simulink model "TrimPlane"  (R2021a)
settings: Solver=ode23t  StartTime=0.0  StopTime=5000  RelTol=1e-3
undefined symbols (not defined in the file or in its folder): F, MIL, Moderate, plane
libraries: aerolibasang x2, shared6dof x1, sharedtransform x1, aerolibadyn x1, aerolibwind2 x1, aerolibatmos2 x1
settings Model: Creator=janbe  LastModifiedBy=janbe

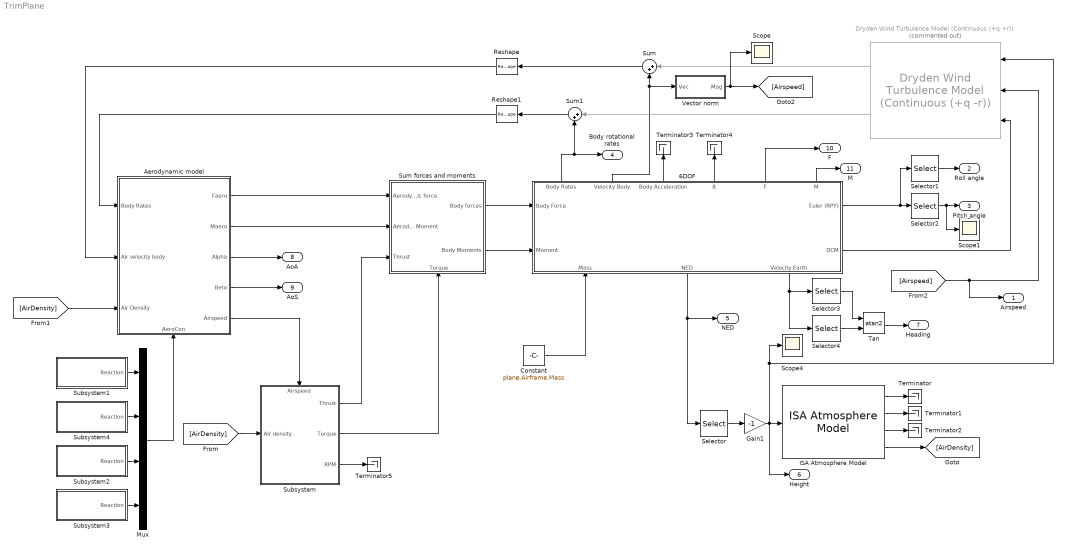
== system TrimPlane ==
  6DOF : Subsystem
      settings: PortSchema="{\"entries\":[{\"content\":{\"sides\":[{\"content\":{\"connectorIds\":[\"In1\",\"In2\"]},\"type\":\"ConnectorPlacement.EquallySpacedRectSide\",\"uuid\":\"48c1bbec-9b7a-4998-8085-77477050d4c3\"},{\"content\":{\"connectorIds\":[\"Out1\",\"Out2\"],\"side\":\"RIGHT\"},\"type\":\"ConnectorPlacement.EquallySpacedRectSide\",\"uuid\":\"5fc5dd37-324a-470e-bd5f-bf29eb3f91cd\"},{\"content\":{\"connectorIds\":[\"Out5\",\"Out6\",\"Out7\",\"Out8\",\"Out9\",\"Out10\"],\"side\":\"TOP\"},\"type\":\"ConnectorPlacement.EquallySpacedRectSide\",\"uuid\":\"ad20a820-91fa-4a98-9c09-942563c80c3d\"},{\"content\":{\"connectorIds\":[\"In3\",\"Out3\",\"Out4\"],\"side\":\"BOTTOM\"},\"type\":\"ConnectorPlacement.EquallySpacedRectSide\",\"uuid\":\"0b972b14-3415-44ab-ae5c-f6c492f3b9a5\"}]},\"type\":\"ConnectorPlacement.EquallySpacedConnector\",\"uuid\":\"3b00a1ae-2557-41be-80c2-23bcdc8281c3\"}],\"packageUris\":[\"http://schema.mathworks.com/mf0/Connector/R2020b\"],\"version\":\"1.0\"}"
  Aerodynamic model : Subsystem
      settings: PortSchema="{\"entries\":[{\"content\":{\"sides\":[{\"content\":{\"connectorIds\":[\"In1\",\"In2\",\"In3\"]},\"type\":\"ConnectorPlacement.EquallySpacedRectSide\",\"uuid\":\"123ed6f9-c03c-44a2-9337-b402a98582dd\"},{\"content\":{\"connectorIds\":[\"Out1\",\"Out2\",\"Out3\",\"Out4\",\"Out5\"],\"side\":\"RIGHT\"},\"type\":\"ConnectorPlacement.EquallySpacedRectSide\",\"uuid\":\"6aca0a3c-b214-45a7-a9f0-b8fb94350ea4\"},{\"content\":{\"connectorIds\":[],\"side\":\"TOP\"},\"type\":\"ConnectorPlacement.EquallySpacedRectSide\",\"uuid\":\"093f64cd-11d7-4128-9556-c22df5842c81\"},{\"content\":{\"connectorIds\":[\"In4\"],\"side\":\"BOTTOM\"},\"type\":\"ConnectorPlacement.EquallySpacedRectSide\",\"uuid\":\"6978f55d-1ae4-4dbf-af4a-386a3019c4ac\"}]},\"type\":\"ConnectorPlacement.EquallySpacedConnector\",\"uuid\":\"655dc0fe-ac89-4e4b-af89-368bfcff1c7c\"}],\"packageUris\":[\"http://schema.mathworks.com/mf0/Connector/R2020b\"],\"version\":\"1.0\"}"
  Constant : Constant  Value=plane.Airframe.Mass
  Dryden Wind Turbulence Model (Continuous (+q +r)) : aerolibwind2/Dryden Wind Turbulence Model  (Continuous (+q -r))  Commented=on  units=Metric (MKS)  spec=MIL-F-8785C  model=Continuous Von Karman (+q -r)  W20=15  Wdeg=0  TurbProb=10^-3 - Moderate  L_high=533.4  Wingspan=19.478  ts=0.1  Seed=[23341 23342 23343 23344]  T_on=off
  Gain1 : Gain  Gain=-1
  ISA Atmosphere Model : aerolibatmos2/ISA Atmosphere Model  custom=off  g=9.80665  gamma=1.4  R=287.0531  L=0.0065  h_trop=11000  h_strat=20000  rho0=1.225  P0=101325  T0=288.15  h0=0
  Mux : Mux
  Reshape : Reshape  OutputDimensionality=Column vector (2-D)
  Reshape1 : Reshape  OutputDimensionality=Column vector (2-D)
  Scope : Scope
  Scope1 : Scope
  Scope4 : Scope
  Selector : Selector  InputPortWidth=3  IndexOptions=Index vector (dialog)  Indices=3  OutputSizes=1
  Selector1 : Selector  InputPortWidth=3  IndexOptions=Index vector (dialog)  Indices=1  OutputSizes=1
  Selector2 : Selector  InputPortWidth=3  IndexOptions=Index vector (dialog)  Indices=2  OutputSizes=1
  Selector3 : Selector  InputPortWidth=3  IndexOptions=Index vector (dialog)  Indices=2  OutputSizes=1
  Selector4 : Selector  InputPortWidth=3  IndexOptions=Index vector (dialog)  Indices=1  OutputSizes=1
  Subsystem : Subsystem
      settings: PortSchema="{\"entries\":[{\"content\":{\"sides\":[{\"content\":{\"connectorIds\":[\"In1\"]},\"type\":\"ConnectorPlacement.EquallySpacedRectSide\",\"uuid\":\"8b318bb3-5013-4f5e-bd3e-2f5669bf6358\"},{\"content\":{\"connectorIds\":[\"Out1\",\"Out2\",\"Out3\"],\"side\":\"RIGHT\"},\"type\":\"ConnectorPlacement.EquallySpacedRectSide\",\"uuid\":\"500402ef-b296-45ac-a743-b1e2b9e33679\"},{\"content\":{\"connectorIds\":[\"In2\"],\"side\":\"TOP\"},\"type\":\"ConnectorPlacement.EquallySpacedRectSide\",\"uuid\":\"5cfe175c-55a3-4920-8fe6-6fd8cc9eed8d\"}]},\"type\":\"ConnectorPlacement.EquallySpacedConnector\",\"uuid\":\"49d65523-413b-4dcb-9879-1a0370ab7ce2\"}],\"packageUris\":[\"http://schema.mathworks.com/mf0/Connector/R2020b\"],\"version\":\"1.0\"}"
  Subsystem1 : Subsystem
  Subsystem2 : Subsystem
  Subsystem3 : Subsystem
  Subsystem4 : Subsystem
  Sum : Sum  Inputs=|++
  Sum forces and moments : Subsystem
      settings: PortSchema="{\"entries\":[{\"content\":{\"sides\":[{\"content\":{\"connectorIds\":[\"In1\",\"In2\",\"In3\"]},\"type\":\"ConnectorPlacement.EquallySpacedRectSide\",\"uuid\":\"38dc5884-e381-4ee1-b666-063f48dc30b0\"},{\"content\":{\"connectorIds\":[\"Out1\",\"Out2\"],\"side\":\"RIGHT\"},\"type\":\"ConnectorPlacement.EquallySpacedRectSide\",\"uuid\":\"f2accc80-19db-41a7-90ee-23d63e2eaee3\"},{\"content\":{\"connectorIds\":[],\"side\":\"TOP\"},\"type\":\"ConnectorPlacement.EquallySpacedRectSide\",\"uuid\":\"1b11c4b8-c720-481f-9c75-f8744fb4ebda\"},{\"content\":{\"connectorIds\":[\"In4\"],\"side\":\"BOTTOM\"},\"type\":\"ConnectorPlacement.EquallySpacedRectSide\",\"uuid\":\"feccc13e-1f0d-4c40-950e-b0861e641184\"}]},\"type\":\"ConnectorPlacement.EquallySpacedConnector\",\"uuid\":\"fb9299ee-4c49-45c5-85b3-a138e0bb7e95\"}],\"packageUris\":[\"http://schema.mathworks.com/mf0/Connector/R2020b\"],\"version\":\"1.0\"}"
  Sum1 : Sum  Inputs=|++
  Tan : Trigonometry  Operator=atan2
  Terminator{,1..5} (6 alike) : Terminator
  Vector norm : Subsystem  mask(Vector norm-2){}
      mask help: Compute the 2-norm (magnitude) of a vector, |v| = sqrt(v'v).
      mask Help:
      | The block compute the 2-norm (or magnitude) of a vector.
      | <P><B>Input:</B> nx1 vector;</P>
      | <P><B>Output:</B> scalar magnitude.</P>
  Airspeed : Outport  Unit=m/s
  Roll angle : Outport  Port=2  Unit=rad
  Pitch angle : Outport  Port=3  Unit=rad
  Body rotational rates : Outport  Port=4  Unit=rad/s
  NED : Outport  Port=5  Unit=m
  Height : Outport  Port=6  Unit=m
  Heading : Outport  Port=7  Unit=rad
  AoA : Outport  Port=8  Unit=rad
  AoS : Outport  Port=9  Unit=rad
  F : Outport  Port=10
  M : Outport  Port=11
  wires:
  Aerodynamic model/2(Maero) -> Sum forces and moments/2(Aerodynamic Moment)
  6DOF/3(NED) -> Selector/1, NED/1
  Subsystem1/1(Reaction) -> Mux/1
  [AirDensity] -> Aerodynamic model/3(Air Density)
  [AirDensity] -> Subsystem/1(Air density)
  Selector2/1 -> Scope1/1, Pitch angle/1
  ISA Atmosphere Model/1 -> Terminator/1
  6DOF/2(DCM) -> Dryden Wind Turbulence Model (Continuous (+q +r))/3
  Dryden Wind Turbulence Model (Continuous (+q +r))/1 -> Sum/1
  Selector4/1 -> Tan/2
  Selector1/1 -> Roll angle/1
  ISA Atmosphere Model/4 -> [AirDensity]
  Vector norm/1(Mag) -> Scope/1, [Airspeed]
  Subsystem/3(RPM) -> Terminator5/1
  Aerodynamic model/4(Beta) -> AoS/1
  Tan/1 -> Heading/1
  Sum1/1 -> Reshape1/1
  Reshape1/1 -> Aerodynamic model/1(Body Rates)
  Constant/1 -> 6DOF/3(Mass)
  Subsystem4/1(Reaction) -> Mux/2
  6DOF/5(Body Rates) -> Body rotational rates/1, Sum1/2
  Subsystem2/1(Reaction) -> Mux/3
  6DOF/1(Euler (RPY)) -> Selector2/1, Selector1/1
  Sum/1 -> Reshape/1
  ISA Atmosphere Model/2 -> Terminator1/1
  Selector3/1 -> Tan/1
  Reshape/1 -> Aerodynamic model/2(Air velocity body)
  6DOF/6(Velocity Body) -> Vector norm/1(Vec), Sum/2
  Selector/1 -> Gain1/1
  Aerodynamic model/1(Faero) -> Sum forces and moments/1(Aerodynamic force)
  Aerodynamic model/3(Alpha) -> AoA/1
  Sum forces and moments/1(Body forces) -> 6DOF/1(Body Force)
  6DOF/4(Velocity Earth) -> Selector4/1, Selector3/1
  Sum forces and moments/2(Body Moments) -> 6DOF/2(Moment)
  Subsystem3/1(Reaction) -> Mux/4
  Dryden Wind Turbulence Model (Continuous (+q +r))/2 -> Sum1/1
  Mux/1 -> Aerodynamic model/4(AeroCon)
  Gain1/1 -> Height/1, Scope4/1, Dryden Wind Turbulence Model (Continuous (+q +r))/1, ISA Atmosphere Model/1
  [Airspeed] -> Airspeed/1, Dryden Wind Turbulence Model (Continuous (+q +r))/2
  ISA Atmosphere Model/3 -> Terminator2/1
  6DOF/8(Inertial Acceleration) -> Terminator4/1
  6DOF/7(Body Acceleration) -> Terminator3/1
  Aerodynamic model/5(Airspeed) -> Subsystem/2(Airspeed)
  Subsystem/1(Thrust) -> Sum forces and moments/3(Thrust)
  Subsystem/2(Torque) -> Sum forces and moments/4(Torque)
  6DOF/10(M) -> M/1
  6DOF/9(F) -> F/1

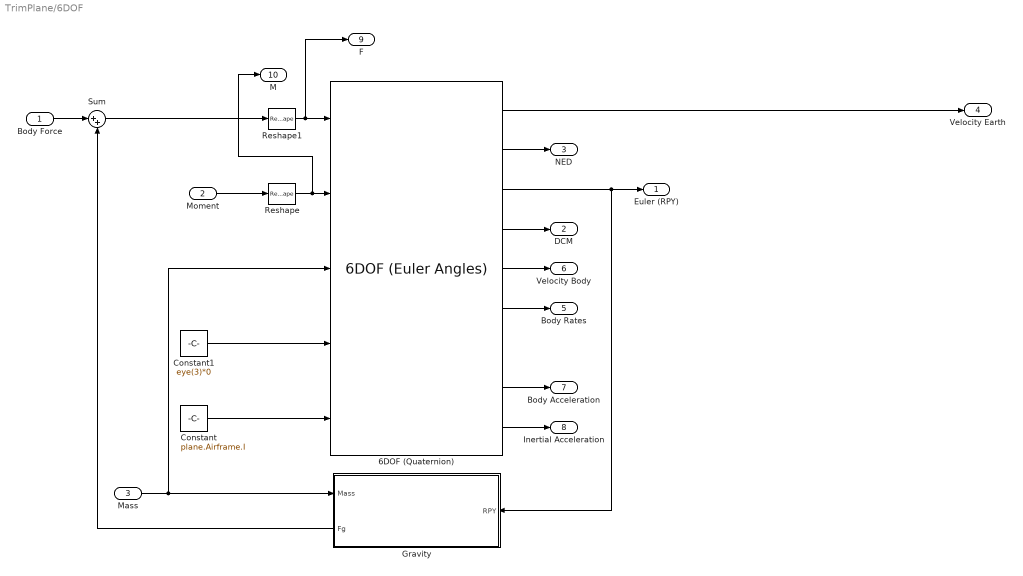
== system TrimPlane/6DOF ==
  Body Force : Inport  Unit=N  PortDimensions=[3 1]
  Moment : Inport  Port=2  Unit=N*m  PortDimensions=[3 1]
  Mass : Inport  Port=3  Unit=kg  PortDimensions=1
  6DOF (Quaternion) : shared6dof/6DOF (Euler Angles)  units=Metric (MKS)  mtype=Custom Variable  rep=Quaternion  xme_0=[0 0 -plane.trim.height]  Vm_0=plane.trim.BodyV  eul_0=[plane.trim.roll plane.trim.pitch 0]  pm_0=plane.trim.BodyRate  mass_0=1.0  mass_e=0.5  mass_f=2.0  inertia=eye(3)  inertia_e=eye(3)  inertia_f=2*eye(3)  k_quat=1.0  vre_flag=off  abi_flag=on  aMode=0  xme_statename=['North','East','Down']  Vm_statename=['Vx','Vy','Vz']  eul_statename=''  quat_statename=''  pm_statename=['Roll_rate_p','Pitch_rate_q','Yaw_rate_r']  mass_statename=''
      settings: SourceProductBaseCode=AE,PW,DR,MT,UV,VE
  Constant : Constant  Value=plane.Airframe.I
  Constant1 : Constant  Value=eye(3)*0
  Gravity : Subsystem
      settings: PortSchema="{\"entries\":[{\"content\":{\"sides\":[{\"content\":{\"connectorIds\":[\"In1\"]},\"type\":\"ConnectorPlacement.EquallySpacedRectSide\",\"uuid\":\"6f94d740-82bf-458e-8aa5-36b62f7e3ce2\"},{\"content\":{\"connectorIds\":[\"In2\",\"Out1\"],\"side\":\"RIGHT\"},\"type\":\"ConnectorPlacement.EquallySpacedRectSide\",\"uuid\":\"bdd5df12-d14f-445f-9bdc-a906ddbef1d8\"},{\"content\":{\"connectorIds\":[],\"side\":\"TOP\"},\"type\":\"ConnectorPlacement.EquallySpacedRectSide\",\"uuid\":\"cebee685-71c6-4366-9c39-37a9487371f5\"},{\"content\":{\"connectorIds\":[],\"side\":\"BOTTOM\"},\"type\":\"ConnectorPlacement.EquallySpacedRectSide\",\"uuid\":\"d1e10f76-8344-46b9-aae8-e8382cc28aaf\"}]},\"type\":\"ConnectorPlacement.EquallySpacedConnector\",\"uuid\":\"3d57e629-d59a-436c-b4c0-fcf54e0e0441\"}],\"packageUris\":[\"http://schema.mathworks.com/mf0/Connector/R2020b\"],\"version\":\"1.0\"}"
  Reshape : Reshape
  Reshape1 : Reshape
  Sum : Sum  Inputs=|++
  Euler (RPY) : Outport  Unit=rad
  DCM : Outport  Port=2
  NED : Outport  Port=3  Unit=m
  Velocity Earth : Outport  Port=4  Unit=m/s
  Body Rates : Outport  Port=5  Unit=rad/s
  Velocity Body : Outport  Port=6  Unit=m/s
  Body Acceleration : Outport  Port=7  Unit=m/s^2
  Inertial Acceleration : Outport  Port=8  Unit=m/s^2
  F : Outport  Port=9
  M : Outport  Port=10
  wires:
  6DOF (Quaternion)/5 -> Velocity Body/1
  6DOF (Quaternion)/3 -> Gravity/1(RPY), Euler (RPY)/1
  6DOF (Quaternion)/6 -> Body Rates/1
  6DOF (Quaternion)/8 -> Body Acceleration/1
  6DOF (Quaternion)/9 -> Inertial Acceleration/1
  6DOF (Quaternion)/1 -> Velocity Earth/1
  Mass/1 -> Gravity/2(Mass), 6DOF (Quaternion)/3
  Constant1/1 -> 6DOF (Quaternion)/4
  Reshape/1 -> M/1, 6DOF (Quaternion)/2
  Reshape1/1 -> F/1, 6DOF (Quaternion)/1
  6DOF (Quaternion)/2 -> NED/1
  Body Force/1 -> Sum/1
  Gravity/1(Fg) -> Sum/2
  Moment/1 -> Reshape/1
  Constant/1 -> 6DOF (Quaternion)/5
  Sum/1 -> Reshape1/1
  6DOF (Quaternion)/4 -> DCM/1

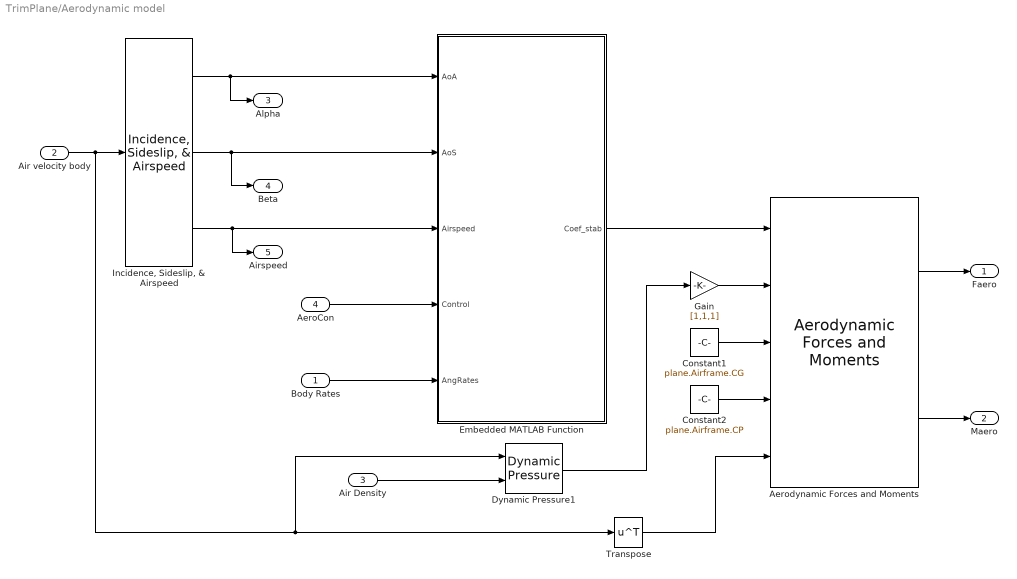
== system TrimPlane/Aerodynamic model ==
  Body Rates : Inport  Unit=rad/s  PortDimensions=[3 1]
  Air velocity body : Inport  Port=2  Unit=m/s  PortDimensions=[3 1]
  Air Density : Inport  Port=3  Unit=kg/m^3  PortDimensions=1
  AeroCon : Inport  Port=4  Unit=rad
  "Aerodynamic Forces and Moments " : aerolibadyn/Aerodynamic Forces and Moments   inputAxes=Stability  outputForceAxes=Body  outputMomentAxes=Body  S=plane.Airframe.A  b=plane.Airframe.S  cbar=plane.Airframe.MAC
  Constant1 : Constant  Value=plane.Airframe.CG
  Constant2 : Constant  Value=plane.Airframe.CP
  Dynamic Pressure1 : aerolibasang/Dynamic Pressure
  Embedded MATLAB Function : MATLAB Function  TreatAsAtomicUnit=on  mask{CL0=plane.Aerodynamic.CL0, dCLdAoA=plane.Aerodynamic.dCLdAoA, CD0=plane.Aerodynamic.CD0, CDmin=plane.Aerodynamic.CDmin, dCDdCL=plane.Aerodynamic.dCDdCL, dClAoS=plane.Aerodynamic.dClAoS, dClY=plane.Aerodynamic.dClY, dClP=plane.Aerodynamic.dClP, Cm0=plane.Aerodynamic.Cm0, dCmCL=plane.Aerodynamic.dCmCL, dCmQ=plane.Aerodynamic.dCmQ, dCnAoS=plane.Aerodynamic.CnAoS, dCnY=plane.Aerodynamic.dCnY, dCnP=plane.Aerodynamic.dCnP, C2M=plane.Aerodynamic.C2M, C2CL=plane.Aerodynamic.C2CL, C2CD=plane.Aerodynamic.C2CD}
  Gain : Gain  Gain=[1,1,1]
  "Incidence, Sideslip, & Airspeed" : aerolibasang/Incidence, Sideslip, & Airspeed
  Transpose : Math  Operator=transpose  SaturateOnIntegerOverflow=on
  Faero : Outport  Unit=N
  Maero : Outport  Port=2  Unit=N*m
  Alpha : Outport  Port=3  Unit=rad
  Beta : Outport  Port=4  Unit=rad  PortDimensions=1
  Airspeed : Outport  Port=5  Unit=m/s
  wires:
  Body Rates/1 -> Embedded MATLAB Function/5(AngRates)
  Air Density/1 -> Dynamic Pressure1/2
  AeroCon/1 -> Embedded MATLAB Function/4(Control)
  "Incidence, Sideslip, & Airspeed"/3 -> Airspeed/1, Embedded MATLAB Function/3(Airspeed)
  "Incidence, Sideslip, & Airspeed"/1 -> Alpha/1, Embedded MATLAB Function/1(AoA)
  "Incidence, Sideslip, & Airspeed"/2 -> Beta/1, Embedded MATLAB Function/2(AoS)
  "Aerodynamic Forces and Moments "/1 -> Faero/1
  Dynamic Pressure1/1 -> Gain/1
  Constant2/1 -> "Aerodynamic Forces and Moments "/4
  Constant1/1 -> "Aerodynamic Forces and Moments "/3
  Transpose/1 -> "Aerodynamic Forces and Moments "/5
  Gain/1 -> "Aerodynamic Forces and Moments "/2
  Embedded MATLAB Function/1(Coef_stab) -> "Aerodynamic Forces and Moments "/1
  "Aerodynamic Forces and Moments "/2 -> Maero/1
  Air velocity body/1 -> "Incidence, Sideslip, & Airspeed"/1, Dynamic Pressure1/1, Transpose/1

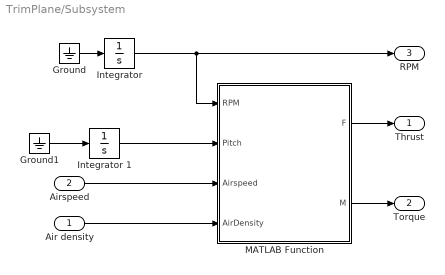
== system TrimPlane/Subsystem ==
  Air density : Inport  Unit=kg/m^3
  Airspeed : Inport  Port=2  Unit=m/s
  Ground : Ground
  Ground1 : Ground
  "Integrator " : Integrator  InitialCondition=plane.trim.Engine_RPM  LimitOutput=on  UpperSaturationLimit=plane.powertrain.SpeedSat(1)  LowerSaturationLimit=plane.powertrain.SpeedSat(2)  ContinuousStateAttributes='Engine_RPM'
  Integrator 1 : Integrator  InitialCondition=plane.trim.Engine_Pitch  LimitOutput=on  UpperSaturationLimit=max(plane.powertrain.pitch)  LowerSaturationLimit=min(plane.powertrain.pitch)  ContinuousStateAttributes='Engine_pitch'
  MATLAB Function : MATLAB Function  TreatAsAtomicUnit=on  mask{D=plane.powertrain.D, J2cT=plane.powertrain.J2cT, PitchVec=plane.powertrain.pitch, L=plane.powertrain.L}
      mask prompts: D "Propeller diameter"; J2cT "Propeller J to cT dependency for range of pitch angles"; PitchVec "considered pitch angles"; L "Engine position"
  Thrust : Outport  Unit=N
  Torque : Outport  Port=2  Unit=N*m
  RPM : Outport  Port=3  Unit=rpm
  wires:
  "Integrator "/1 -> MATLAB Function/1(RPM), RPM/1
  Airspeed/1 -> MATLAB Function/3(Airspeed)
  MATLAB Function/1(F) -> Thrust/1
  Air density/1 -> MATLAB Function/4(AirDensity)
  MATLAB Function/2(M) -> Torque/1
  Ground/1 -> "Integrator "/1
  Ground1/1 -> Integrator 1/1
  Integrator 1/1 -> MATLAB Function/2(Pitch)

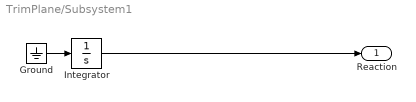
== system TrimPlane/Subsystem1 ==
  Ground : Ground
  "Integrator " : Integrator  InitialCondition=plane.trim.AileronL  LimitOutput=on  UpperSaturationLimit=plane.ailerons.DeflectionSat(1)  LowerSaturationLimit=plane.ailerons.DeflectionSat(2)  ContinuousStateAttributes='AileronL'
  Reaction : Outport  Unit=rad
  wires:
  "Integrator "/1 -> Reaction/1
  Ground/1 -> "Integrator "/1

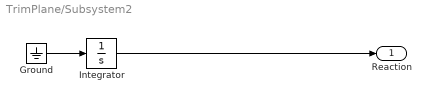
== system TrimPlane/Subsystem2 ==
  Ground : Ground
  "Integrator " : Integrator  InitialCondition=plane.trim.Elevator  LimitOutput=on  UpperSaturationLimit=plane.elevator.DeflectionSat(1)  LowerSaturationLimit=plane.elevator.DeflectionSat(2)  ContinuousStateAttributes='Elevator'
  Reaction : Outport  Unit=rad
  wires:
  "Integrator "/1 -> Reaction/1
  Ground/1 -> "Integrator "/1

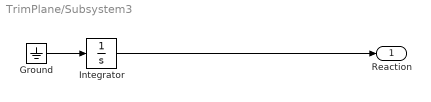
== system TrimPlane/Subsystem3 ==
  Ground : Ground
  "Integrator " : Integrator  InitialCondition=plane.trim.Rudder  LimitOutput=on  UpperSaturationLimit=plane.rudder.DeflectionSat(1)  LowerSaturationLimit=plane.rudder.DeflectionSat(2)  ContinuousStateAttributes='Rudder'
  Reaction : Outport  Unit=rad
  wires:
  "Integrator "/1 -> Reaction/1
  Ground/1 -> "Integrator "/1

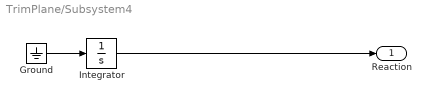
== system TrimPlane/Subsystem4 ==
  Ground : Ground
  "Integrator " : Integrator  InitialCondition=plane.trim.AileronR  LimitOutput=on  UpperSaturationLimit=plane.ailerons.DeflectionSat(1)  LowerSaturationLimit=plane.ailerons.DeflectionSat(2)  ContinuousStateAttributes='AileronR'
  Reaction : Outport  Unit=rad
  wires:
  "Integrator "/1 -> Reaction/1
  Ground/1 -> "Integrator "/1

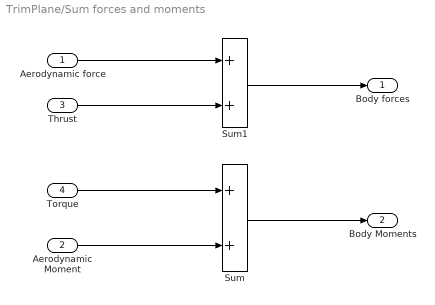
== system TrimPlane/Sum forces and moments ==
  Aerodynamic force : Inport  Unit=N
  Aerodynamic Moment : Inport  Port=2
  Thrust : Inport  Port=3  Unit=N
  Torque : Inport  Port=4
  Sum : Sum
  Sum1 : Sum
  Body forces : Outport  Unit=N
  Body Moments : Outport  Port=2
  wires:
  Sum1/1 -> Body forces/1
  Aerodynamic Moment/1 -> Sum/2
  Sum/1 -> Body Moments/1
  Torque/1 -> Sum/1
  Thrust/1 -> Sum1/2
  Aerodynamic force/1 -> Sum1/1

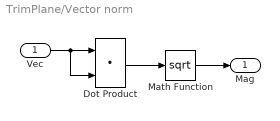
== system TrimPlane/Vector norm ==
  Vec : Inport
  Dot Product : DotProduct  InputSameDT=on  OutDataTypeStr=Inherit: Inherit via internal rule
  Math Function : Math  Operator=sqrt  SignedPower=on  SaturateOnIntegerOverflow=on
  Mag : Outport
  wires:
  Dot Product/1 -> Math Function/1
  Vec/1 -> Dot Product/1, Dot Product/2
  Math Function/1 -> Mag/1

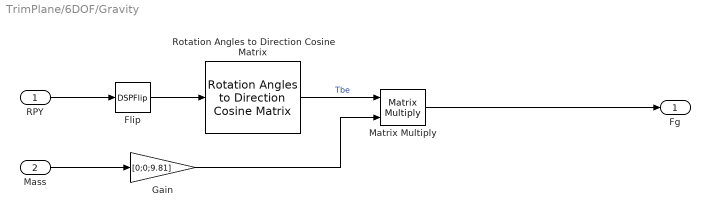
== system TrimPlane/6DOF/Gravity ==
  RPY : Inport
  Mass : Inport  Port=2
  Flip : DSPFlip
  Gain : Gain  Gain=[0;0;9.81]
  Matrix Multiply : Product  Multiplication=Matrix(*)
  Rotation Angles to Direction Cosine Matrix : sharedtransform/Rotation Angles to Direction Cosine Matrix  rotationOrder=ZYX  aMode=aMode
      settings: SourceProductBaseCode=AE,PW,DR,MT,UV,VE
  Fg : Outport
  wires:
  RPY/1 -> Flip/1
  Flip/1 -> Rotation Angles to Direction Cosine Matrix/1
  Mass/1 -> Gain/1
  Rotation Angles to Direction Cosine Matrix/1 -> Matrix Multiply/1  "Tbe"
  Matrix Multiply/1 -> Fg/1
  Gain/1 -> Matrix Multiply/2

== matlab function TrimPlane/Subsystem/MATLAB Function ==
  data: RPM input; Pitch input; F output; Airspeed input; AirDensity input; PitchVec parameter; D parameter; J2cT parameter; L parameter; M output
function [F,M] = ThrustCalculation(RPM,Pitch, Airspeed,AirDensity, PitchVec, D, J2cT,L)
n = RPM./60;
J = Airspeed./(n.*D');
cT_vec = J2cT*[J.^2,J,ones(size(J))]';
cT = zeros(size(J));
for i = 1:length(cT)
    cT(i) = interp1(PitchVec,cT_vec(:,i),Pitch(i),'spline');
end
F_vec = cT.* (n.^2)*AirDensity*D.^4;
F = [sum(F_vec);0;0];
M = L*F_vec;
end

== matlab function TrimPlane/Aerodynamic model/Embedded MATLAB Function ==
  data: AoA input; AoS input; Airspeed input; Coef_stab output; Control input; AngRates input; CL0 parameter; dCLdAoA parameter; CDmin parameter; CD0 parameter; dCDdCL parameter; dClAoS parameter; dClY parameter; dClP parameter; dCmCL parameter; Cm0 parameter; dCmQ parameter; dCnAoS parameter; dCnY parameter; dCnP parameter; C2M parameter; C2CL parameter; C2CD parameter
function Coef_stab  = AeroCoefM(AoA,AoS,Airspeed,Control,AngRates,CL0, dCLdAoA, CDmin, CD0, dCDdCL, dClAoS, dClY, dClP, dCmCL, Cm0, dCmQ, dCnAoS, dCnY, dCnP,C2M, C2CL,C2CD)

    p = AngRates(1);q = AngRates(2); y=AngRates(3);
    %% LIFT
    CL = CL0 + dCLdAoA*AoA;

    %% DRAG
    CD = CD0 + dCDdCL*(CL - CDmin)^2;
    %% Efect of stall
    CL = CL*exp(min(1,((-abs(AoA)+deg2rad(10))))/2-1/2);
    %% ROLLING MOMENT
    %b/(2*Airspeed) * 
    Cl = dClAoS*AoS ;
    dCldPR = dClP*p + dClY*y;
    l = Cl + dCldPR/Airspeed;
     %% PITCHING MOMENT
    Cm = dCmCL*CL + Cm0;
    dCmdQ = dCmQ*q;
    m = Cm + dCmdQ/Airspeed; 
    %% YAWING MOMENT
    % b/(2*Airspeed) * 
    Cn = dCnAoS*AoS;
    dCndPR =  dCnP*p + dCnY*y; 
    n = Cn + dCndPR/Airspeed;
    % Control influence
    CM = C2M*Control;
    CCL = C2CL*Control;
    CCD = C2CD*abs(Control);
    Coef_stab = zeros(6,1);
    Coef_stab = [CD+CCD,0,CL+CCL,l+CM(1),m+CM(2),n+CM(3)]';
end
